simulink subsystem "RackandPinion1"  (R2023a)
settings: Solver=VariableStepAuto  StartTime=0.0  StopTime=10.0  RelTol=1e-3
model mask{J_RackAndPinion=1e-06, i_RackAndPinion=20000, m=0.3}
  mask prompts: J_RackAndPinion "Момент инерции шестерни, кг*м^2"; i_RackAndPinion "Передаточное соотношение зубчатой передачи, рад/м"; m "Масса, кг"
settings Model: Creator=stude  LastModifiedBy=mehra

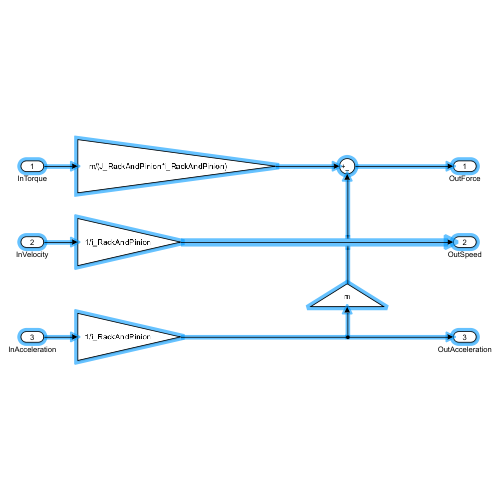
[thumbnail: Simulink's stored preview of the top-level diagram]
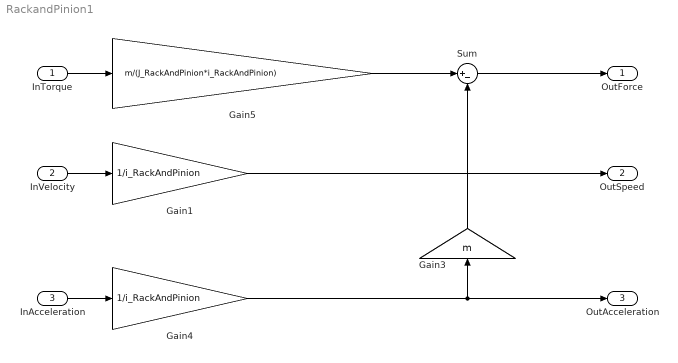
== system RackandPinion1 ==
  InTorque : Inport
  InVelocity : Inport  Port=2
  InAcceleration : Inport  Port=3
  Gain1 : Gain  Gain=1/i_RackAndPinion
  Gain3 : Gain  Gain=m
  Gain4 : Gain  Gain=1/i_RackAndPinion
  Gain5 : Gain  Gain=m/(J_RackAndPinion*i_RackAndPinion)
  Sum : Sum  Inputs=|+-
  OutForce : Outport
  OutSpeed : Outport  Port=2
  OutAcceleration : Outport  Port=3
  wires:
  Gain5/1 -> Sum/1
  InAcceleration/1 -> Gain4/1
  InTorque/1 -> Gain5/1
  Gain4/1 -> OutAcceleration/1, Gain3/1
  Sum/1 -> OutForce/1
  InVelocity/1 -> Gain1/1
  Gain3/1 -> Sum/2
  Gain1/1 -> OutSpeed/1
